simulink model "PID0"  (R2020b)
settings: Solver=ode45  StartTime=0.0  StopTime=10.0  RelTol=1e-3
undefined symbols (not defined in the file or in its folder): Kd, Ki, Kp, N, Ts
settings Model: DataDictionary=problem4.sldd  OrderedModelArguments=off  Creator=DELL  LastModifiedBy=DELL
settings DataIOCC: SaveOutput=off  SaveTime=off

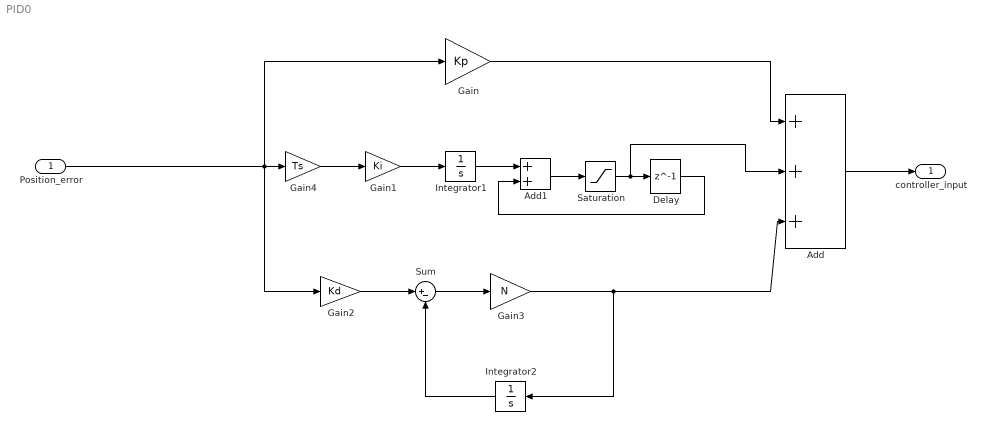
== system PID0 ==
  Position_error : Inport  OutDataTypeStr=double  PortDimensions=1  SampleTime=0
  Add : Sum  Inputs=+++
  Add1 : Sum
  Delay : Delay  DelayLength=1
  Gain : Gain  Gain=Kp
  Gain1 : Gain  Gain=Ki
  Gain2 : Gain  Gain=Kd
  Gain3 : Gain  Gain=N
  Gain4 : Gain  Gain=Ts
  Integrator1 : Integrator
  Integrator2 : Integrator
  Saturation : Saturate  UpperLimit=1  LowerLimit=-1
  Sum : Sum  Inputs=|+-
  controller_input : Outport  OutDataTypeStr=double  PortDimensions=1  SampleTime=0
  wires:
  Gain/1 -> Add/1
  Position_error/1 -> Gain/1, Gain4/1, Gain2/1
  Add/1 -> controller_input/1
  Gain1/1 -> Integrator1/1
  Gain2/1 -> Sum/1
  Sum/1 -> Gain3/1
  Gain3/1 -> Add/3, Integrator2/1
  Integrator2/1 -> Sum/2
  Gain4/1 -> Gain1/1
  Integrator1/1 -> Add1/1
  Add1/1 -> Saturation/1
  Saturation/1 -> Add/2, Delay/1
  Delay/1 -> Add1/2
